simulink model "anav_real"  (R2018a)
settings: Solver=VariableStepAuto  StartTime=0.0  StopTime=inf  RelTol=1e-3
InitFcn:
  | run('initialize.m')
values from neighbouring files (symbols this model uses):
  allObstacles = [1 2 3 4 5 6 7 8 9 10 11 12 ... (3348 elements, 186x3x6)]    [a.mat]    (also in initArena.m = vertcat(limit, obstacle1, obstacle2, obstacle3, obstacle4, o)
  visualObjects = [0 1 2 3 4 5 6 7 8 9 10 11 ... (1164 elements, 194x3x2)]    [a.mat]
settings Model: SnapshotBufferSize=5  SnapshotInterval=1  Creator=alex  LastModifiedBy=hal

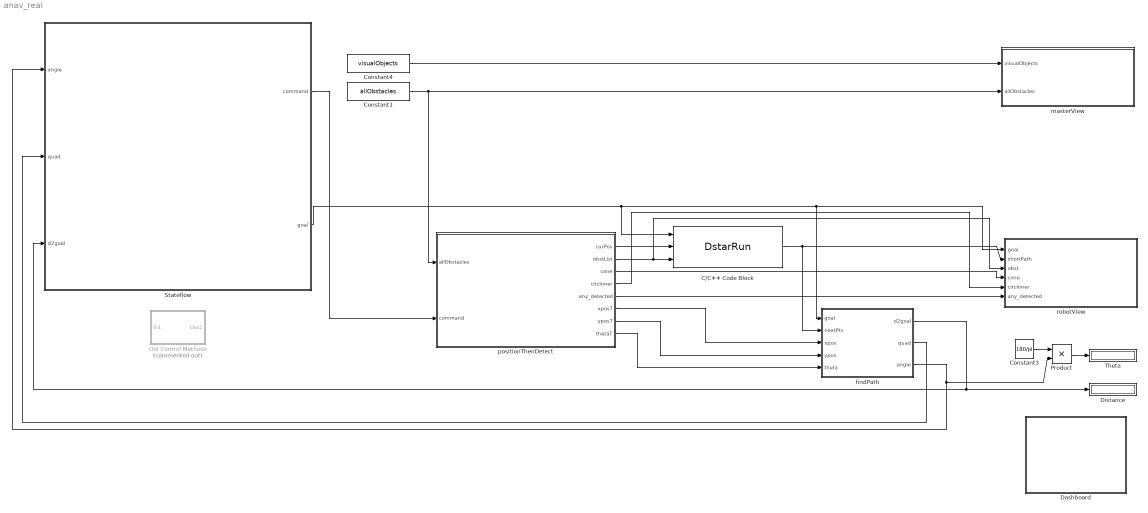
== system anav_real ==
  C/C++ Code Block : S-Function  InitFcn=try, set_param(gcb,'FunctionName','DstarRun'), end  FunctionName=DstarRun  SFunctionModules=DstarRun_wrapper Dstar  SFunctionDeploymentMode=off  EnableBusSupport=off  mask(S-Function Builder){}
      mask help: Simulink:masks:SFunctionBuilder_MD
      mask init:
      | val = [[.9  0.75 0.75 1 1 .9 .9 1]',[1 1 0.75 0.75 .9 .9 1 .9]'];try , sys = get_param(gcb,'SfunBuilderFcnName');if isempty(sys), sys = get_param(gcb,'FunctionName'); end,catch, sys = get_param(gcb,'FunctionName'); end
      settings: CopyFcn=set_param(gcbh,'LinkStatus','none')  PreSaveFcn=try, set_param(gcb,'FunctionName','DstarRun'), end  OpenFcn=sfunctionwizard(gcbh)
      mask Display: plot(val(:,1),val(:,2)),disp(sys), port_label('input',1,'goal'), port_label('input',2,'start'), port_label('input',3,'obst'), port_label('output',1,'shortPath')
  Constant1 : Constant  Value=allObstacles
  Constant3 : Constant  Value=180/pi
  Constant4 : Constant  Value=visualObjects
  Dashboard : Subsystem
  "Distance " : Display
  "Old Control Methods " : Subsystem  Commented=on
  Product : Product
  Stateflow : Stateflow chart  TreatAsAtomicUnit=on
  Theta : Display
  findPath : MATLAB Function  TreatAsAtomicUnit=on
  masterView : MATLAB Function  TreatAsAtomicUnit=on
  positionThenDetect : MATLAB Function  TreatAsAtomicUnit=on
  robotView : MATLAB Function  TreatAsAtomicUnit=on
  wires:
  Constant1/1 -> positionThenDetect/1(allObstacles), masterView/2(allObstacles)
  Stateflow/1(command) -> positionThenDetect/2(command)
  positionThenDetect/5(any_detected) -> robotView/6(any_detected)
  findPath/3(angle) -> Stateflow/1(angle), Product/2
  Product/1 -> Theta/1
  findPath/2(quad) -> Stateflow/2(quad)
  positionThenDetect/3(cone) -> robotView/4(cone)
  positionThenDetect/4(circInner) -> robotView/5(circInner)
  C/C++ Code Block/1 -> findPath/2(nextPts), robotView/2(shortPath)
  positionThenDetect/1(curPos) -> C/C++ Code Block/2
  positionThenDetect/2(obstList) -> robotView/3(obst), C/C++ Code Block/3
  Constant3/1 -> Product/1
  positionThenDetect/6(xposT) -> findPath/3(xpos)
  positionThenDetect/7(yposT) -> findPath/4(ypos)
  positionThenDetect/8(thetaT) -> findPath/5(theta)
  Constant4/1 -> masterView/1(visualObjects)
  Stateflow/2(goal) -> robotView/1(goal), findPath/1(goal), C/C++ Code Block/1
  findPath/1(d2goal) -> Stateflow/3(d2goal), "Distance "/1

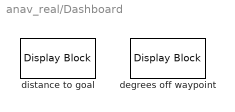
== system anav_real/Dashboard ==
  "degrees off waypoint " : DisplayBlock  WebBlockId=71  LabelPosition=Hide
  distance to goal : DisplayBlock  WebBlockId=70  LabelPosition=Hide

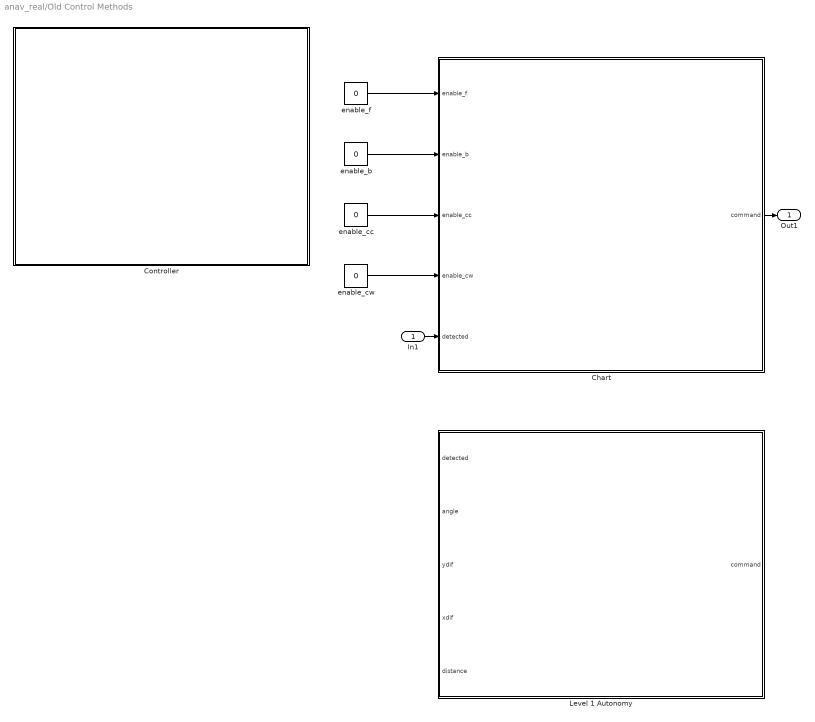
== system anav_real/Old Control Methods  ==
  In1 : Inport
  Chart : Stateflow chart  TreatAsAtomicUnit=on
  Controller : Subsystem
  "Level 1 Autonomy " : Stateflow chart  TreatAsAtomicUnit=on
  "enable_b " : Constant  Value=0
  "enable_cc " : Constant  Value=0
  "enable_cw " : Constant  Value=0
  "enable_f " : Constant  Value=0
  Out1 : Outport
  wires:
  Chart/1(command) -> Out1/1
  "enable_cw "/1 -> Chart/4(enable_cw)
  "enable_cc "/1 -> Chart/3(enable_cc)
  "enable_b "/1 -> Chart/2(enable_b)
  In1/1 -> Chart/5(detected)
  "enable_f "/1 -> Chart/1(enable_f)

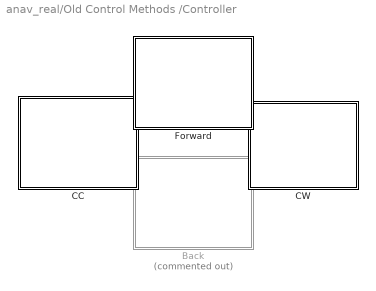
== system anav_real/Old Control Methods /Controller ==
  Back : Subsystem  Commented=on  DialogController=hmiCreateDDGDialog  IsWebBlock=on  mask(MWDashboardBlock){webBlockId=1a5e94ef-030e-49cd-b944-b929b04abc70, webBlockType=pushbutton, ShowInLibBrwoser=on, ShowInitialText=on, HMISrcModelName=anav_real}
      mask prompts: webBlockId "WebBlock Id"; webBlockType "WebBlock Type"; HMISrcModelName "Source Model"
      mask help: SimulinkHMI:dialogs:PushButtonDialogDesc
      mask Help: helpview([docroot '/mapfiles/simulink.map'], 'hmi_push_button')
      mask Display:
      | model = bdroot(gcb);
      | if strcmp(get_param(model,'BlockDiagramType'), 'library')
      |     image([(matlabroot) '/toolbox/simulink/hmi/icons/PushButton.png']);
      | end
  "CC " : Subsystem  DialogController=hmiCreateDDGDialog  IsWebBlock=on  mask(MWDashboardBlock){webBlockId=f6d6ee6b-2047-45ee-ab2e-570b521bf019, webBlockType=pushbutton, ShowInLibBrwoser=on, ShowInitialText=on, HMISrcModelName=anav_real}
      mask prompts: webBlockId "WebBlock Id"; webBlockType "WebBlock Type"; HMISrcModelName "Source Model"
      mask help: SimulinkHMI:dialogs:PushButtonDialogDesc
      mask Help: helpview([docroot '/mapfiles/simulink.map'], 'hmi_push_button')
      mask Display:
      | model = bdroot(gcb);
      | if strcmp(get_param(model,'BlockDiagramType'), 'library')
      |     image([(matlabroot) '/toolbox/simulink/hmi/icons/PushButton.png']);
      | end
  "CW " : Subsystem  DialogController=hmiCreateDDGDialog  IsWebBlock=on  mask(MWDashboardBlock){webBlockId=5b3cd59d-fae2-469c-adcb-5a1af564bf62, webBlockType=pushbutton, ShowInLibBrwoser=on, ShowInitialText=on, HMISrcModelName=anav_real}
      mask prompts: webBlockId "WebBlock Id"; webBlockType "WebBlock Type"; HMISrcModelName "Source Model"
      mask help: SimulinkHMI:dialogs:PushButtonDialogDesc
      mask Help: helpview([docroot '/mapfiles/simulink.map'], 'hmi_push_button')
      mask Display:
      | model = bdroot(gcb);
      | if strcmp(get_param(model,'BlockDiagramType'), 'library')
      |     image([(matlabroot) '/toolbox/simulink/hmi/icons/PushButton.png']);
      | end
  Forward : Subsystem  DialogController=hmiCreateDDGDialog  IsWebBlock=on  mask(MWDashboardBlock){webBlockId=418d2ee9-92ed-471b-995b-1589f387356b, webBlockType=pushbutton, ShowInLibBrwoser=on, ShowInitialText=on, HMISrcModelName=anav_real}
      mask prompts: webBlockId "WebBlock Id"; webBlockType "WebBlock Type"; HMISrcModelName "Source Model"
      mask help: SimulinkHMI:dialogs:PushButtonDialogDesc
      mask Help: helpview([docroot '/mapfiles/simulink.map'], 'hmi_push_button')
      mask Display:
      | model = bdroot(gcb);
      | if strcmp(get_param(model,'BlockDiagramType'), 'library')
      |     image([(matlabroot) '/toolbox/simulink/hmi/icons/PushButton.png']);
      | end

== system anav_real/Old Control Methods /Controller/Back ==

== system anav_real/Old Control Methods /Controller/CC  ==

== system anav_real/Old Control Methods /Controller/CW  ==

== system anav_real/Old Control Methods /Controller/Forward ==

== stateflow chart anav_real/Stateflow ==
  settings: stateMachineType=MOORE_MACHINE
  state change_goal
    state to_bin
      goal = bin
      dir = b
    state to_mine
      goal = mine
      dir = f
    state to_home_out
      goal = home_out
      dir = f
    state to_home_in
      goal = home_in
      dir = f
    (junction 345) -> to_bin [order 2] : [goal(2) == home_in(2)]
    (junction 345) -> to_mine [order 3] : [goal(2) == home_out(2)]
    (junction 345) -> to_home_in [order 1] : [goal(2) == mine(2)]
    (junction 345) -> to_home_out [order 4] : [goal(2) == bin(2)]
  state end
    command = 0
  state ideal_path
    state forward_ideal
      command = 1
    state cc_to_ideal
      command = 3
    state cw_to_ideal
      command = 4
    state backwards_ideal
      command = 2
    forward_ideal -> (junction 243) [order 3]
    (junction 265) -> cc_to_ideal [order 1] : [angle>=0]
    (junction 243) -> (junction 265) [order 2] : [(dir == f & (quad == 2 | quad == 3))...
        | | (dir == b & (quad == 1 | quad == 4)) ]
    (junction 265) -> cw_to_ideal [order 2] : [angle<0]
    (junction 261) -> cc_to_ideal [order 2] : [angle<0]
    (junction 243) -> (junction 261) [order 1] : [(dir == f & (quad == 1 | quad == 4))...
        | | (dir == b & (quad == 2 | quad == 3)) ]
    backwards_ideal -> (junction 243) [order 3]
    (junction 261) -> cw_to_ideal [order 1] : [angle>=0]
  state goal_reached
    stage = stage + 1
    command = 0
  state temp
  state start
    mine = [50 30]
    home_in = [7 15]
    home_out = [7 14]
    bin = [7 7]
    f = 0
    b = pi
    %%%%%%%%%
    stage = 1
    dir = f
    goal = mine
  to_bin -> (junction 361)
  to_mine -> (junction 361)
  (junction 283) -> (junction 345) [order 2]
  to_home_out -> (junction 361)
  (junction 361) -> (junction 394)
  to_home_in -> (junction 361)
  (junction 283) -> end [order 1] : [stage > 12]
  (junction 375) -> (junction 211) [order 1] : [(dir == f & (quad == 2 | quad == 3))...
      | | (dir == b & (quad == 1 | quad == 4)) ]
  (junction 211) -> (junction 161) : [(angle < pi & angle > pi-pi/128)...
      | | (angle > -pi & angle < -pi+pi/128)]
  goal_reached -> (junction 283)
  (junction 375) -> (junction 209) [order 2] : [(dir == f & (quad == 1 | quad == 4))...
      | | (dir == b & (quad == 2 | quad == 3)) ]
  (junction 209) -> (junction 161) : [(angle > -pi/128 & angle < pi/128)]
  (junction 183) -> (junction 375)
  (junction 161) -> temp
  forward_ideal -> (junction 183) [order 2]
  temp -> (junction 382)
  (junction 377) -> goal_reached : [d2goal <= 0.5]
  forward_ideal -> (junction 377) [order 1]
  (junction 382) -> forward_ideal [order 1] : [dir == f]
  cc_to_ideal -> (junction 183)
  cw_to_ideal -> (junction 183)
  (junction 394) -> (junction 243)
  (junction 382) -> backwards_ideal [order 2] : [dir == b]
  backwards_ideal -> (junction 183) [order 2]
  backwards_ideal -> (junction 377) [order 1]
  (default) -> start
  start -> (junction 394)
  data: command output; angle input; quad input; goal output; d2goal input; mine local double size=[1 2]; home_in local double size=[1 2]; bin local double size=[1 2]; home_out local double size=[1 2]; dir local double size=1; f local double size=1; b local double size=1; stage local double size=1

== matlab function anav_real/positionThenDetect ==
  data: curPos output size=[1 2]; obstList output size=[2052 2]; cone output size=[4 3]; circInner output size=[2 100]; allObstacles input; command input; any_detected output size=1; xposT output size=1; yposT output size=1; thetaT output size=1
function [curPos, obstList, cone, circInner, any_detected, xposT, yposT, thetaT] = positionThenDetect(allObstacles, command)
    persistent xpos ypos theta occupancyMap
    xmax = 57; % Physical wall just outside these distances 
    ymax = 36; 
    obstList = zeros(xmax*ymax,2);
    
    % Define start location
    if isempty(xpos)
        occupancyMap = logical(zeros(ymax, xmax));
        xpos = 3;
        ypos = ymax-3;
        theta = pi/2;
    end
        
    % Robot specifications 
    botRadius = 0.5; % Used for graphic circle and Dstar inflation 
    coneDepth = 6;
    speed = 0.5;
    turnSpeed = pi/128;

    % Radius of robot vision and representing circles 
    r = sqrt(botRadius^2+(2*coneDepth^2)-2*botRadius*sqrt(2*coneDepth^2)*cos(135*pi/180));
    t = linspace(-pi,pi);
    xc = [r*cos(t); botRadius*cos(t)];
    yc = [-r*sin(t); -botRadius*sin(t)];

    % Update position and rotation based on command (send to motor
    % controlers)
    if command == 1 % forward
        xpos = xpos + speed*cos(theta);
        ypos = ypos + speed*sin(theta);
    elseif command == 2 % back
        xpos = xpos - speed*cos(theta);
        ypos = ypos - speed*sin(theta);
    elseif command == 3 % counter clockwise
        theta = theta + turnSpeed;
    elseif command == 4 % clockwise 
        theta = theta - turnSpeed;
    end

    % Calculate rotated cone around origin (not necissary)
    thigh = theta + asin(coneDepth/r);
    tlow = thigh-2*asin(coneDepth/r);
    x = [botRadius*cos(theta) r*cos(thigh) r*cos(tlow) botRadius*cos(theta)];
    y = [botRadius*sin(theta) r*sin(thigh) r*sin(tlow) botRadius*sin(theta)];
    z = zeros(1,4);
    rotated_cone = fliplr(rot90(vertcat(x,y,z),3));
        
    % Translate cone to new position (not necissary)
    cone = rotated_cone;
    cone(:,1) = rotated_cone(:,1) + xpos;
    cone(:,2) = rotated_cone(:,2) + ypos;
    cone(:,3) = rotated_cone(:,3);
    
    % Translate circle to new position (not necissary)
    circInner = zeros(2, length(t));
    circInner(1,:) = xc(2,:) + xpos;
    circInner(2,:) = yc(2,:) + ypos;
    
    % Create current position variable for D* start value 
    curPos = horzcat(xpos, ypos);

    % Check if obstacle is in vision cone (get data from sensors)
    allObstList = vertcat(allObstacles(:,:,1), allObstacles(:,:,2), allObstacles(:,:,3), allObstacles(:,:,4), allObstacles(:,:,5), allObstacles(:,:,6));
    detected = detectRotated(allObstList, cone);
  
    % Create a list of obstacles that are detected 
    allObstX = allObstList(:,1);
    allObstY = allObstList(:,2);
    if any(detected)
        x = allObstX(detected==1);
        y = allObstY(detected==1);
        
        % Convert list of x,y coordinates to occupancy map 
        occupancyMapNew = createOccupancyMap(x, y, xmax, ymax);
        occupancyMap = occupancyMap | occupancyMapNew;
    end
    
    % Convert complete occupancy map back to list  
    i = 0;
    for r = 1:ymax
        for c = 1:xmax
            i = i+1;
            cur = occupancyMap(r,c);
            if cur == 1
                obstList(i,:) = [c r];
            elseif cur == 0
                obstList(i,:) = [nan nan];
            end
        end
    end
   
    % Indicate if any obstacles are detected 
    any_detected = double(any(detected(:)));
    
    % Assign persistent variables to temporary variable, allows the
    % function to output these values 
    xposT = xpos;
    yposT = ypos;
    thetaT = theta;
end

== stateflow chart anav_real/Old Control Methods /Chart ==
  settings: stateMachineType=MOORE_MACHINE
  state no_input
    command = 0
  state check_detected
  state back
    command = 2
  state counter_clockwise
    command = 3
  state clockwise
    command = 4
  state forward
    command = 1
  (default) -> no_input
  no_input -> check_detected [order 1] : [enable_f == 1]
  forward -> no_input [order 1] : [enable_f == 0]
  check_detected -> no_input [order 2] : [detected==1]
  no_input -> back [order 4] : [enable_b ==1]
  back -> no_input : [enable_b== 0]
  no_input -> counter_clockwise [order 3] : [enable_cc == 1]
  counter_clockwise -> no_input : [enable_cc == 0]
  no_input -> clockwise [order 2] : [enable_cw == 1]
  clockwise -> no_input : [enable_cw == 0]
  forward -> check_detected [order 2] : [detected==1]
  check_detected -> forward [order 1] : [detected==0]
  data: enable_f input; enable_b input; enable_cc input; enable_cw input; command output; detected input

== matlab function anav_real/masterView ==
  data: visualObjects input; allObstacles input
function masterView(visualObjects, allObstacles)   
    % Visualize data
    plot(visualObjects(:,1,1), visualObjects(:,2,1), 'k-');
    hold on 
    grid on
    grid minor
    xlim([0 58]);
    ylim([0 37]);
    xlabel('Field Length (x10 cm)')
    ylabel('Field Width (x10 cm)')
    title('2D Autonomous Navigation With Object Avoidance')
    plot(visualObjects(:,1,2), visualObjects(:,2,2), 'k-');
    for i = 1:size(allObstacles,3)
        plot(allObstacles(:,1,i), allObstacles(:,2,i), 'k-');
    end
end

== matlab function anav_real/robotView ==
  data: goal input; shortPath input; obst input; cone input; circInner input; any_detected input
function robotView(goal, shortPath, obst, cone, circInner, any_detected)
    if any_detected
        coneColor = 'r';
    else
        coneColor = 'k';
    end
    
    coneFig = plot(cone(:,1),cone(:,2), coneColor);
    circOFig = plot(circInner(1,:),circInner(2,:));
    shortPathFig = plot(shortPath(:,1), shortPath(:,2), 'g-');
    plot(obst(:,1), obst(:,2), 'r*');
    plot(goal(1), goal(2), 'g*');
    set([coneFig circOFig shortPathFig],'LineWidth', 2)
    hold off
end

== matlab function anav_real/findPath ==
  data: goal input; nextPts input; d2goal output; xpos input; ypos input; theta input; quad output; angle output
function [d2goal, quad, angle] = findPath(goal, nextPts, xpos, ypos, theta)
    % Calculate intantaneous angle/dist between current and ideal orientation 
    [d2waypoint, xdif, ydif] = distFromPath(nextPts(3,:), xpos, ypos);
    angle = degFromPath(nextPts(3,:), xpos, ypos, theta); 
    
    % Calculate distance from current goal
    d2goal = distFromPath(goal, xpos, ypos);
    d2goal = d2goal(1);
    
    % Calculate quadrant of endPt as if robot is the origin 
    quad = 0;
    if xdif >= 0 && ydif >= 0
        quad = 1;
    elseif xdif < 0 && ydif >= 0
        quad = 2;
    elseif xdif < 0 && ydif < 0
        quad = 3;
    elseif xdif >= 0 && ydif < 0
        quad = 4;
    end
end

== stateflow chart anav_real/Old Control Methods /Level 1 Autonomy  ==
  settings: stateMachineType=MOORE_MACHINE
  state diversion
    state turn_until_clear
      command = 4
    state forward_diversion
      command = 1
    state turn_opposite_until_touch
      command = 3
    forward_diversion -> turn_until_clear [order 2] : [detected == 1]
    turn_until_clear -> forward_diversion [order 2] : [detected == 0]
    turn_opposite_until_touch -> turn_until_clear [order 2] : [detected == 1]
    forward_diversion -> turn_opposite_until_touch [order 3]
  state ideal_path
    state forward_ideal_path
      command = 1
    state turn_to_ideal
      command = 3
    forward_ideal_path -> turn_to_ideal [order 3]
  state start
    %goal = [25 30]
  state arrive_mining_zone
    state arrived_mining_area
      command = 0
  turn_until_clear -> (junction 183) [order 1]
  (junction 206) -> (junction 211) [order 2] : [[(xdif < 0 & ydif > 0) | (xdif < 0 & ydif < 0)]]
  (junction 211) -> (junction 161) : [(angle < pi & angle > pi-pi/128) | (angle > -pi & angle < -pi+pi/128)]
  (junction 161) -> turn_until_clear [order 2]
  (junction 183) -> (junction 206)
  (junction 209) -> (junction 161) : [(angle > -pi/128 & angle < pi/128)]
  (junction 206) -> (junction 209) [order 1] : [(xdif > 0 & ydif > 0) | (xdif > 0 & ydif < 0)]
  forward_ideal_path -> (junction 183) [order 2]
  turn_to_ideal -> (junction 183)
  turn_opposite_until_touch -> (junction 183) [order 1]
  (junction 161) -> forward_ideal_path [order 1] : [detected == 0]
  forward_ideal_path -> (junction 200) [order 1]
  start -> turn_to_ideal
  forward_diversion -> (junction 200) [order 1]
  (junction 200) -> arrived_mining_area : [distance < 3]
  (default) -> start
  data: command output; detected input; angle input; ydif input; xdif input; distance input
